simulink model "Sub2_2023"  (R2023b)
settings: Solver=FixedStepDiscrete  StartTime=0.0  StopTime=4.5  FixedStep=7.5e-05  RelTol=1e-3  EnableMultiTasking=on
undefined symbols (not defined in the file or in its folder): D1, D11, Delta
libraries: spsSeriesRLCBranchLib x41, spsLoadFlowBusLib x29, spsDistributedParametersLineLib x19, spsThreePhaseSeriesRLCLoadLib x15, spsThreePhaseTransformerTwoWindingsLib x13, spsThreePhaseParallelRLCLoadLib x11, spsThreePhaseVIMeasurementLib x11, spsSynchronousMachinepuStandardLib x7, spsExcitationSystemLib x7, spsHydraulicTurbineandGovernorLib x7, spsGenericPowerSystemStabilizerLib x7, spsMultiBandPowerSystemStabilizerLib x7
(part 3 of 5)

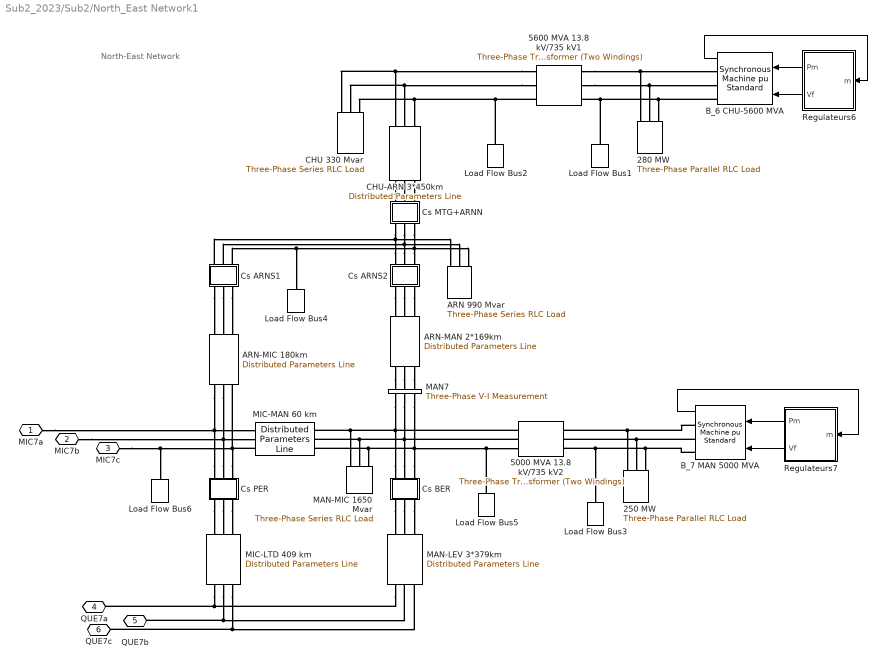
== system Sub2_2023/Sub2/North_East Network1 ==
  note: North-East Network
  250 MW : spsThreePhaseParallelRLCLoadLib/Three-Phase Parallel RLC Load  LConnTagsString=A|B|C  Configuration=Y (grounded)  NominalVoltage=(13800)*1  Vabc=[1e3 1e3 1e3]  Vabcp=[1e3 1e3 1e3]  NominalFrequency=60  UnbalancedPower=off  ActivePower=250000000  InductivePower=0  CapacitivePower=0  Pabc=[10e3 9e3 11e3]  QLabc=[100 90 110]  QCabc=[100 90 110]  Pabcp=[10e3 9e3 11e3]  QLabcp=[100 90 110]  QCabcp=[100 90 110]  Measurements=None  LoadType=constant PQ
  280 MW : spsThreePhaseParallelRLCLoadLib/Three-Phase Parallel RLC Load  LConnTagsString=A|B|C  Configuration=Y (grounded)  NominalVoltage=(13800)*1  Vabc=[1e3 1e3 1e3]  Vabcp=[1e3 1e3 1e3]  NominalFrequency=60  UnbalancedPower=off  ActivePower=280000000  InductivePower=0  CapacitivePower=0  Pabc=[10e3 9e3 11e3]  QLabc=[100 90 110]  QCabc=[100 90 110]  Pabcp=[10e3 9e3 11e3]  QLabcp=[100 90 110]  QCabcp=[100 90 110]  Measurements=None  LoadType=constant PQ
  5000 MVA 13.8 kV/735 kV2 : spsThreePhaseTransformerTwoWindingsLib/Three-Phase Transformer (Two Windings)  Winding1Connection=Delta (D1)  Winding2Connection=Yg  CoreType=Three single-phase transformers  SetSaturation=off  Hysteresis=off  DataFile='basic_model'  SetInitialFlux=off  Measurements=None  UNITS=pu  NominalPower=[ 5000e6 60 ]  Winding1="[ 13.8e3 0.002  0.0]"  Winding2=[ 735e3 0.002 0.12]  Rm=500  Lm=500  L0=0.5  Saturation="[ 0,0  ;  0.005,1.2  ;  1.0,1.4 ]"  InitialFluxes=[ 0.8 , -0.8 , 0.7 ]  BreakLoop=off  DiscreteSolver=Trapezoidal iterative  DataType=off  TransfoNumber=0
  5600 MVA 13.8 kV/735 kV1 : spsThreePhaseTransformerTwoWindingsLib/Three-Phase Transformer (Two Windings)  Winding1Connection=Delta (D1)  Winding2Connection=Yg  CoreType=Three single-phase transformers  SetSaturation=off  Hysteresis=off  DataFile='basic_model'  SetInitialFlux=off  Measurements=None  UNITS=pu  NominalPower=[ 5600e6 60 ]  Winding1="[ 13.8e3 0.002  0.0]"  Winding2=[ 735e3 0.002 0.12]  Rm=500  Lm=500  L0=0.5  Saturation="[ 0,0  ;  0.005,1.2  ;  1.0,1.4 ]"  InitialFluxes=[ 0.8 , -0.8 , 0.7 ]  BreakLoop=off  DiscreteSolver=Trapezoidal iterative  DataType=off  TransfoNumber=0
  ARN 990 Mvar : spsThreePhaseSeriesRLCLoadLib/Three-Phase Series RLC Load  LConnTagsString=A|B|C  Configuration=Y (grounded)  NominalVoltage=735e3  Vabc=[1e3 1e3 1e3]  Vabcp=[1e3 1e3 1e3]  NominalFrequency=60  UnbalancedPower=off  ActivePower=3300000  InductivePower=990e6  CapacitivePower=0  Pabc=[10e3 9e3 11e3]  QLabc=[100 90 110]  QCabc=[100 90 110]  Pabcp=[10e3 9e3 11e3]  QLabcp=[100 90 110]  QCabcp=[100 90 110]  Measurements=None  LoadType=constant Z
  ARN-MAN 2*169km : spsDistributedParametersLineLib/Distributed Parameters Line  Phases=3  Length=169  Frequency=60  Resistance="[0.01273  0.3864]/2"  Inductance="[0.9337e-3  4.1264e-3]/2"  Capacitance=[12.74e-9 7.751e-9]*2  x1=[-0.000975 1.7310716577648e-09 347873.977312542 -681165.145140991;-0.0009 1.66282026610766e-09 366991.883229433 -671058.367402292;-0.000825 1.59323964137178e-09 385816.421450034 -660415.155872229;-0.00075 1.52238540524399e-09 404332.543926518 -649244.018571252;-0.000675 1.45031419751651e-09 422525.449153882 -637553.885535596;-0.0006 1.37708363081009e-09 440380.594002048 -625354.101678744;-0.000525 1.30275224451929e-09 457883.705341419 -612654.419321249;-0.00045 1.227379458017e-09 475020.791452595 -599464.990394876;-0.000375 1.15102552315551e-09 491778.153211146 -585796.358327302;-0.0003 1.07375147610208e-09 508142.395038477 -571659.449613867;-0.000225 9.95619088547613e-10 524100.435610055 -557065.565083093;-0.00015 9.16690818327239e-10 539639.518312411 -542026.370862981;-7.5e-05 8.37029759492534e-10 554747.22144059 -526553.889055283]  x2=[-0.000975 1.53641947846113e-09 232985.418240288 -689450.364519062;-0.0009 1.49169542852533e-09 252383.458947623 -682588.200672253;-0.000825 1.44577894008767e-09 271579.748179473 -675180.386261777;-0.00075 1.39870671808647e-09 290558.940715937 -667232.842981129;-0.000675 1.35051639133576e-09 309305.864880893 -658751.923974807;-0.0006 1.30124648244541e-09 327805.534670003 -649744.408759702;-0.000525 1.25093637702673e-09 346043.16173029 -640217.497805657;-0.00045 1.19962629220823e-09 364004.167181727 -630178.806779522;-0.000375 1.14735724448663e-09 381674.19327137 -619636.360457307;-0.0003 1.09417101693894e-09 399039.114850723 -608598.586309297;-0.000225 1.04011012582169e-09 416085.050667168 -597074.307763262;-0.00015 9.85217786584077e-10 432798.374460424 -585072.737151144;-7.5e-05 9.29537879322206e-10 449165.725855173 -572603.46834486]  x3=[-0.000975 -3.38800758696293e-12 1583.75858462532 -1421.24992657805;-0.0009 -3.62113287945408e-12 1623.30400424475 -1375.90902523865;-0.000825 -3.85136349372659e-12 1661.55177948058 -1329.46824327658;-0.00075 -4.07851538695005e-12 1698.47133564649 -1281.96470474239;-0.000675 -4.30240697737656e-12 1734.03315981417 -1233.43638323794;-0.0006 -4.52285928949439e-12 1768.20882440548 -1183.92207156094;-0.000525 -4.73969609709827e-12 1800.97100991707 -1133.46135069455;-0.00045 -4.95274406416191e-12 1832.29352675911 -1082.09455816696;-0.000375 -5.16183288340019e-12 1862.15133619089 -1029.86275580616;-0.0003 -5.36679541241016e-12 1890.52057033639 -976.80769691581;-0.000225 -5.56746780728218e-12 1917.3785512639 -922.9717928982;-0.00015 -5.76368965357417e-12 1942.70380911441 -868.39807935129;-7.5e-05 -5.9553040945445e-12 1966.47609926427 -813.130181666682]  x4=[-0.000975 1.03362527745804e-11 1569.30174481215 -9115.59279820568;-0.0009 1.01548326150274e-11 1826.37892659032 -9067.58416140718;-0.000825 9.96529483765609e-12 2081.9961289991 -9012.32703656874;-0.00075 9.76779095606568e-12 2335.94901555798 -8949.86559539049;-0.000675 9.56247885183719e-12 2588.03458021503 -8880.24976859283;-0.0006 9.34952264832539e-12 2838.05130962692 -8803.53520600253;-0.000525 9.129092579461e-12 3085.79934424553 -8719.78323206715;-0.00045 8.90136485366839e-12 3331.08063808267 -8629.06079683322;-0.000375 8.66652151300721e-12 3573.69911702496 -8531.44042242736;-0.0003 8.42475028765076e-12 3813.46083557254 -8427.00014508323;-0.000225 8.17624444581736e-12 4050.17413187606 -8315.82345276054;-0.00015 7.92120263927471e-12 4283.64978094831 -8197.99921840608;-7.5e-05 7.65982874454068e-12 4513.70114592771 -8073.62162891002]  x5=0.000955765248222805  V1=ones(3,3)  V2=ones(3,3)  I1=ones(3,3)  I2=ones(3,3)  nHarmo=1  Measurements=None  Decoupling=on  VsMag0=[624500.542746028 624501.9043063 624500.043262054]  VrMag0=[594207.380493384 594208.101305747 594207.286862453]  VsAngle0=[18.1135948354144 -101.886530201481 138.113424134237]  VrAngle0=[9.73160889878888 -110.268441654022 129.731523430542]  IsMag0=[1744.35611857347 1744.39210598435 1744.37536737855]  IrMag0=[7582.44376493454 7582.43378992783 7582.40838117123]  IsAngle0=[39.1559168024549 -80.8440356055105 159.154916919419]  IrAngle0=[0.828149284031303 -119.172115933983 120.828081951977]
      settings: AttributesFormatString=\n  LibrarySourceBlock=sps_lib/Power Grid Elements/Distributed Parameters Line
  ARN-MIC 180km : spsDistributedParametersLineLib/Distributed Parameters Line  Phases=3  Length=180  Frequency=60  Resistance="[0.01273  0.3864]"  Inductance="[0.9337e-3  4.1264e-3]"  Capacitance=[12.74e-9 7.751e-9]  x1=[-0.00105 1.17550663706793e-09 336203.730988142 -674396.627298138;-0.000975 1.11045162417448e-09 355134.952563357 -664622.476598413;-0.0009 1.04450893324313e-09 373782.28469124 -654317.036859961;-0.000825 9.7773127785208e-10 392130.820979802 -643488.546093628;-0.00075 9.10172039037302e-10 410165.893889875 -632145.660429254;-0.000675 8.41885222620616e-10 427873.086460121 -620297.447196085;-0.0006 7.72925416038243e-10 445238.243831729 -607953.377674497;-0.000525 7.03347744704445e-10 462247.484563591 -595123.319524794;-0.00045 6.33207827945111e-10 478887.211728917 -581817.528899156;-0.000375 5.62561734536522e-10 495144.123784406 -568046.642243022;-0.0003 4.91465937884828e-10 511005.225203302 -553821.667792484;-0.000225 4.19977270882071e-10 526457.836863812 -539153.976774469;-0.00015 3.48152880474837e-10 541489.606184609 -524055.294316752;-7.5e-05 2.7605018198187e-10 556088.51699929 -508537.690075074]  x2=[-0.00105 4.32054145383614e-09 192165.57848684 -719334.039085178;-0.000975 4.26552520912623e-09 212424.764832694 -713613.931123558;-0.0009 4.20709916882887e-09 232514.142071749 -707323.371104057;-0.000825 4.14531003782672e-09 252417.651063218 -700467.387604106;-0.00075 4.08020720940571e-09 272119.381246546 -693051.461192015;-0.000675 4.01184272577075e-09 291603.583360071 -685081.520045889;-0.0006 3.94027123644407e-09 310854.682030743 -676563.935214738;-0.000525 3.86554995457915e-09 329857.288224836 -667505.515525552;-0.00045 3.78773861122544e-09 348596.211549708 -657913.502140431;-0.000375 3.70689940758025e-09 367056.472396768 -647795.562768113;-0.0003 3.62309696526611e-09 385223.313915946 -637159.785534523;-0.000225 3.53639827467318e-09 403082.213812094 -626014.672517248;-0.00015 3.44687264140818e-09 420618.895953885 -614369.132949109;-7.5e-05 3.35459163089256e-09 437819.341785936 -602232.476096253]  x3=[-0.00105 3.17397778533418e-12 149.001660749432 -364.5409355399;-0.000975 3.41695138621498e-12 159.247423691846 -360.183291874008;-0.0009 3.65719352843875e-12 169.365886680328 -355.537723195582;-0.000825 3.89451216611283e-12 179.348961170383 -350.607943101142;-0.00075 4.12871759034934e-12 189.188666845009 -345.397892381469;-0.000675 4.35962258091563e-12 198.877137994043 -339.91173587139;-0.0006 4.5870425558952e-12 208.406629801887 -334.153859120481;-0.000525 4.81079571923969e-12 217.769524538595 -328.128864887315;-0.00045 5.03070320609386e-12 226.958337649373 -321.841569460099;-0.000375 5.24658922577742e-12 235.965723737613 -315.296998806598;-0.0003 5.45828120230941e-12 244.784482436694 -308.500384556456;-0.000225 5.66560991236276e-12 253.407564165843 -301.457159819114;-0.00015 5.86840962053892e-12 261.828075765464 -294.172954840662;-7.5e-05 6.06651821185409e-12 270.039286007422 -286.653592503108]  x4=[-0.00105 3.98244780356522e-12 1187.65933351944 -4979.4651542716;-0.000975 3.61607808742167e-12 1327.95758028664 -4943.89904376789;-0.0009 3.24681773378287e-12 1467.19427808259 -4904.3808560128;-0.000825 2.87496192372567e-12 1605.25812322147 -4860.94218124095;-0.00075 2.50080791309503e-12 1742.03874957792 -4813.61774366432;-0.000675 2.12465479488231e-12 1877.42681681204 -4762.44537371424;-0.0006 1.74680326013487e-12 2011.3140977744 -4707.46597780026;-0.000525 1.36755535758826e-12 2143.59356502113 -4648.72350561027;-0.00045 9.87214252213096e-13 2274.15947637007 -4586.26491497776;-0.000375 6.06083982869597e-13 2402.9074594294 -4520.14013434441;-0.0003 2.24469219263587e-13 2529.73459503138 -4450.40202284814;-0.000225 -1.57324981601807e-13 2654.53949950433 -4377.10632806823;-0.00015 -5.38993419284062e-13 2777.22240571719 -4300.31164146164;-7.5e-05 -9.20230993873817e-13 2897.68524283186 -4220.07935152584]  x5=0.00101797482059234  V1=ones(3,3)  V2=ones(3,3)  I1=ones(3,3)  I2=ones(3,3)  nHarmo=1  Measurements=None  Decoupling=on  VsMag0=[615273.936100198 615275.237959109 615273.425867188]  VrMag0=[607930.231676026 607930.976808573 607930.152147035]  VsAngle0=[19.1774103741833 -100.822714483785 139.17724295487]  VrAngle0=[7.63692875074031 -112.363120449614 127.636843332411]  IsMag0=[322.896150602072 322.910343515583 322.909058922829]  IrMag0=[4197.50413399039 4197.49907033644 4197.4882687283]  IsAngle0=[14.9112658693506 -105.087543385411 134.909680310663]  IrAngle0=[6.09512812442481 -113.905082032172 126.095082904961]
      settings: AttributesFormatString=\n  LibrarySourceBlock=sps_lib/Power Grid Elements/Distributed Parameters Line
  "B_6 CHU-5600 MVA " : spsSynchronousMachinepuStandardLib/Synchronous Machine pu Standard  PresetModel=No  MechanicalLoad=Mechanical power Pm  ShowDetailedParameters=on  RotorType=Salient-pole  Units=per unit standard parameters  MeasurementBus=off  NominalParameters="[ 5600E6  13800   60 ]"  Reactances1=[ 31 32 33 34 35 36 37 ]  Reactances2=[ 1.305, 0.296, 0.252, 0.474, 0.243, 0.18 ]  dAxisTimeConstants=Short-circuit  qAxisTimeConstants=Open-circuit  TimeConstants1=[]  TimeConstants2=[]  TimeConstants3=[]  TimeConstants4=[]  TimeConstants5=[ 1.01, 0.053, 0.1 ]  TimeConstants6=[]  TimeConstants7=[]  TimeConstants8=[]  StatorResistance=2.8544e-3  Mechanical="[ 4.0 0  32]"  PolePairs=32  InitialConditions=[0 -61.7964 0.894782 0.894782 0.894782 8.48442 -111.516 128.484 1.31361]  SetSaturation=off  Saturation=[0.6404,0.7127,0.8441,0.9214,0.9956,1.082,1.19,1.316,1.457;0.7,0.7698,0.8872,0.9466,0.9969,1.046,1.1,1.151,1.201]  LoadFlowParameters=[1 5000000000 0 0 0]  TsPowergui=0  TsBlock=-1  IterativeModel=Trapezoidal non iterative  IterativeDiscreteModel=Trapezoidal non iterative  BusType=PV  Pref=5000000000  Qref=0  Qmin=-Inf  Qmax=Inf  PLF=0  QLF=0
  B_7 MAN 5000 MVA : spsSynchronousMachinepuStandardLib/Synchronous Machine pu Standard  PresetModel=No  MechanicalLoad=Mechanical power Pm  ShowDetailedParameters=on  RotorType=Salient-pole  Units=per unit standard parameters  MeasurementBus=off  NominalParameters="[ 5000E6  13800   60 ]"  Reactances1=[ 31 32 33 34 35 36 37 ]  Reactances2=[ 1.305, 0.296, 0.252, 0.474, 0.243, 0.18 ]  dAxisTimeConstants=Short-circuit  qAxisTimeConstants=Open-circuit  TimeConstants1=[]  TimeConstants2=[]  TimeConstants3=[]  TimeConstants4=[]  TimeConstants5=[ 1.01, 0.053, 0.1 ]  TimeConstants6=[]  TimeConstants7=[]  TimeConstants8=[]  StatorResistance=2.8544e-3  Mechanical="[ 3.7 0  32]"  PolePairs=32  InitialConditions=[0 -81.9543 0.907703 0.907703 0.907703 -8.76021 -128.76 111.24 1.25655]  SetSaturation=off  Saturation=[0.6404,0.7127,0.8441,0.9214,0.9956,1.082,1.19,1.316,1.457;0.7,0.7698,0.8872,0.9466,0.9969,1.046,1.1,1.151,1.201]  LoadFlowParameters=[1 4500000000 0 0 0]  TsPowergui=0  TsBlock=-1  IterativeModel=Trapezoidal non iterative  IterativeDiscreteModel=Trapezoidal non iterative  BusType=PV  Pref=4500000000  Qref=0  Qmin=-Inf  Qmax=Inf  PLF=0  QLF=0
  CHU 330 Mvar : spsThreePhaseSeriesRLCLoadLib/Three-Phase Series RLC Load  LConnTagsString=A|B|C  Configuration=Y (grounded)  NominalVoltage=735e3  Vabc=[1e3 1e3 1e3]  Vabcp=[1e3 1e3 1e3]  NominalFrequency=60  UnbalancedPower=off  ActivePower=1100000  InductivePower=330e6  CapacitivePower=0  Pabc=[10e3 9e3 11e3]  QLabc=[100 90 110]  QCabc=[100 90 110]  Pabcp=[10e3 9e3 11e3]  QLabcp=[100 90 110]  QCabcp=[100 90 110]  Measurements=None  LoadType=constant Z
  CHU-ARN 3*450km : spsDistributedParametersLineLib/Distributed Parameters Line  Phases=3  Length=450  Frequency=60  Resistance="[0.01273  0.3864]/3"  Inductance="[0.9337e-3  4.1264e-3]/3"  Capacitance=[12.74e-9 7.751e-9]*3  x1=[-0.00255 1.80867377993606e-09 0 0;-0.002475 1.72308488593625e-09 0 0;-0.0024 1.6361185842427e-09 0 0;-0.002325 1.54784439438636e-09 0 0;-0.00225 1.45833288140396e-09 0 0;-0.002175 1.36765559942941e-09 0 0;-0.0021 1.2758850344945e-09 0 0;-0.002025 1.18309454658472e-09 0 0;-0.00195 1.08935831099635e-09 0 0;-0.001875 9.94751259041912e-10 0 0;-0.0018 8.993490181512e-10 0 0;-0.001725 8.03227851415879e-10 0 0;-0.00165 7.06464596625934e-10 0 0;-0.001575 6.09136604846718e-10 336692.12965357 -649852.524072933;-0.0015 5.1132167858569e-10 354929.318552013 -640074.408280607;-0.001425 4.13098009598284e-10 372882.782383807 -629784.626799769;-0.00135 3.14544116382617e-10 390538.16942466 -618991.405124295;-0.001275 2.15738781413e-10 407881.36622831 -607703.37119045;-0.0012 1.16760988162435e-10 424898.508908591 -595929.54847985;-0.001125 1.76898579644369e-11 441575.994222016 -583679.348806222;-0.00105 -8.13954132353542e-11 457900.490441999 -570962.564791752;-0.000975 -1.80415618187197e-10 473858.948016035 -557789.362039008;-0.0009 -2.79291601654312e-10 489438.609997312 -544170.271004713;-0.000825 -3.7794432368837e-10 504627.022242419 -530116.178581862;-0.00075 -4.76294922812813e-10 519412.043366998 -515638.319396901;-0.000675 -5.74264779063516e-10 533781.85445138 -500748.266828946;-0.0006 -6.71775576836382e-10 547724.96848845 -485457.923758193;-0.000525 -7.68749367491635e-10 561230.239566184 -469779.513050943;-0.00045 -8.65108631664776e-10 574286.871777518 -453725.567788827;-0.000375 -9.60776341234369e-10 586884.427850438 -437308.921250055;-0.0003 -1.05567602089715e-09 599012.837491367 -420542.696650687;-0.000225 -1.14973180930121e-09 610662.405435208 -403440.296654135;-0.00015 -1.24286851968841e-09 621823.819195594 -386015.392657282;-7.5e-05 -1.33501169999749e-09 632488.156509137 -368281.913861772]  x2=[-0.00255 2.55703265416158e-09 0 0;-0.002475 2.53163349239611e-09 0 0;-0.0024 2.50421058155211e-09 0 0;-0.002325 2.47478584308493e-09 0 0;-0.00225 2.44338279868027e-09 0 0;-0.002175 2.41002655145137e-09 0 0;-0.0021 2.37474376587187e-09 0 0;-0.002025 2.33756264646073e-09 0 0;-0.00195 2.29851291523592e-09 0 0;-0.001875 2.2576257879551e-09 0 0;-0.0018 2.21493394916222e-09 0 0;-0.001725 2.17047152606001e-09 0 0;-0.00165 2.12427406122919e-09 0 0;-0.001575 2.07637848421631e-09 24661.2186380129 -733238.396737066;-0.0015 2.0268230820128e-09 45380.4401578333 -732248.159297928;-0.001425 1.97564746844896e-09 66063.3852481355 -730672.573884019;-0.00135 1.92289255252726e-09 86693.5202790741 -728512.899994213;-0.001275 1.86860050572032e-09 107254.353836357 -725770.864038773;-0.0012 1.81281472825965e-09 127729.44990423 -722448.657959287;-0.001125 1.75557981444221e-09 148102.441004175 -718548.937476463;-0.00105 1.69694151698237e-09 168357.041278825 -714074.819967188;-0.000975 1.63694671043793e-09 188477.059510626 -709029.881972542;-0.0009 1.5756433537393e-09 208446.412064849 -703418.156338769;-0.000825 1.51308045185183e-09 228249.135746606 -697244.128993477;-0.00075 1.44930801660206e-09 247869.400561575 -690512.73535966;-0.000675 1.38437702669898e-09 267291.522370264 -683229.356410397;-0.0006 1.31833938698243e-09 286499.975425668 -675399.814367378;-0.000525 1.2512478869312e-09 305479.404784313 -667030.368046718;-0.00045 1.18315615846389e-09 324214.638580765 -658127.707855748;-0.000375 1.1141186330664e-09 342690.700155786 -648698.95044481;-0.0003 1.04419049828023e-09 360892.820028447 -638751.633018313;-0.000225 9.73427653586374e-10 378806.447702621 -628293.707309608;-0.00015 9.01886665720188e-10 396417.263298435 -617333.533224497;-7.5e-05 8.29624723452754e-10 413711.188999357 -605879.872158446]  x3=[-0.00255 4.79707758720459e-12 0 0;-0.002475 4.73527209386888e-12 0 0;-0.0024 4.66968129647343e-12 0 0;-0.002325 4.60035762729809e-12 0 0;-0.00225 4.52735650262333e-12 0 0;-0.002175 4.45073627843124e-12 0 0;-0.0021 4.37055820375673e-12 0 0;-0.002025 4.28688637172591e-12 0 0;-0.00195 4.1997876683211e-12 0 0;-0.001875 4.10933171891314e-12 0 0;-0.0018 4.01559083260396e-12 0 0;-0.001725 3.9186399444238e-12 0 0;-0.00165 3.81855655542927e-12 0 0;-0.001575 3.7154206707502e-12 -336.540930617868 -2064.60581281028;-0.0015 3.60931473563478e-12 -278.039507495116 -2073.29664774071;-0.001425 3.50032356954406e-12 -219.315823844219 -2080.33012105345;-0.00135 3.38853429834859e-12 -160.416822479385 -2085.70061029753;-0.001275 3.27403628468133e-12 -101.389586361122 -2089.40382238603;-0.0012 3.15692105650254e-12 -42.2813009588338 -2091.43679702786;-0.001125 3.03728223393369e-12 16.8607834685153 -2091.7979090942;-0.00105 2.91521545441901e-12 75.9893896435381 -2090.4868699176;-0.000975 2.79081829627436e-12 135.057251063157 -2087.50472752271;-0.0009 2.66419020068462e-12 194.01714978272 -2082.85386578852;-0.000825 2.53543239221193e-12 252.82195416131 -2076.53800254276;-0.00075 2.40464779787832e-12 311.424656538048 -2068.56218658987;-0.000675 2.27194096488743e-12 369.778410809307 -2058.93279367507;-0.0006 2.13741797705108e-12 427.836569876765 -2047.65752138774;-0.000525 2.00118636998746e-12 485.552722936382 -2034.74538300803;-0.00045 1.86335504515885e-12 542.880732578489 -2020.20670030178;-0.000375 1.72403418281743e-12 599.774771669327 -2004.05309526952;-0.0003 1.58333515392887e-12 656.189359984554 -1986.29748085593;-0.000225 1.4413704311441e-12 712.079400565444 -1966.95405062752;-0.00015 1.29825349889039e-12 767.400215768702 -1946.03826742645;-7.5e-05 1.1540987626536e-12 822.107582981091 -1923.56685100977]  x4=[-0.00255 1.90509802475781e-11 0 0;-0.002475 1.89178495284245e-11 0 0;-0.0024 1.87695961698107e-11 0 0;-0.002325 1.86063386832032e-11 0 0;-0.00225 1.84282075741389e-11 0 0;-0.002175 1.82353452379009e-11 0 0;-0.0021 1.80279058456898e-11 0 0;-0.002025 1.78060552213818e-11 0 0;-0.00195 1.75699707089717e-11 0 0;-0.001875 1.73198410308064e-11 0 0;-0.0018 1.70558661367235e-11 0 0;-0.001725 1.67782570442144e-11 0 0;-0.00165 1.64872356697402e-11 0 0;-0.001575 1.61830346513347e-11 -291.743024303928 -14207.2379327624;-0.0015 1.58658971626376e-11 110.022151992647 -14209.8063832468;-0.001425 1.55360767185051e-11 511.699378264315 -14201.0157319257;-0.00135 1.51938369723538e-11 912.967559882261 -14180.8730059114;-0.001275 1.48394515054003e-11 1313.50592920171 -14149.3943069907;-0.0012 1.44732036079646e-11 1712.99430197867 -14106.6047987541;-0.001125 1.40953860530121e-11 2111.11333332032 -14052.5386864796;-0.00105 1.37063008621155e-11 2507.54477296443 -13987.2391897902;-0.000975 1.33062590640231e-11 2901.97171968375 -13910.7585081044;-0.0009 1.28955804460276e-11 3294.07887461201 -13823.157778909;-0.000825 1.24745932983325e-11 3683.55279328901 -13724.5070288866;-0.00075 1.20436341516223e-11 4070.0821362233 -13614.8851179372;-0.000675 1.16030475080452e-11 4453.35791777224 -13494.3796761393;-0.0006 1.11531855658227e-11 4833.07375314037 -13363.0870336992;-0.000525 1.06944079377084e-11 5208.92610329875 -13221.1121439465;-0.00045 1.02270813635185e-11 5580.61451762939 -13068.5684994357;-0.000375 9.75157941696631e-12 5947.84187410091 -12905.5780412222;-0.0003 9.26828220703232e-12 6310.3146167833 -12732.2710613846;-0.000225 8.77757607411151e-12 6667.74299051209 -12548.7860988707;-0.00015 8.27985328117847e-12 7019.84127251415 -12355.2698287523;-7.5e-05 7.77551170021847e-12 7366.32800081013 -12151.8769449748]  x5=0.00254493705148084  V1=ones(3,3)  V2=ones(3,3)  I1=ones(3,3)  I2=ones(3,3)  nHarmo=1  Measurements=None  Decoupling=on  VsMag0=[597589.636778476 597591.191031021 597588.179734199]  VrMag0=[599025.218159165 599025.681050673 599025.146419465]  VsAngle0=[31.4089201475902 -88.5913271983155 151.408667420066]  VrAngle0=[5.9463220799337 -114.053711405448 125.946266994119]  IsMag0=[1726.12548309379 1726.16866029094 1726.16794416809]  IrMag0=[11726.067575369 11726.0492062877 11726.0164561764]  IsAngle0=[-5.23898774455876 -125.238187761817 114.760171100695]  IrAngle0=[2.84375678806129 -117.156479810906 122.843716218945]
      settings: AttributesFormatString=\n  LibrarySourceBlock=sps_lib/Power Grid Elements/Distributed Parameters Line
  "Cs ARNS1 " : Subsystem  mask{Xc=25}
      mask prompts: Xc "Condensator Reactance at  60Hz  (ohm):"
      mask help: Series Compensation
      mask init:
      | Cs=1/Xc/(2*pi*60);
      mask Display: disp('Cs')
  Cs ARNS2 : Subsystem  mask{Xc=25/2}
      mask prompts: Xc "Condensator Reactance at  60Hz  (ohm):"
      mask help: Series Compensation
      mask init:
      | Cs=1/Xc/(2*pi*60);
      mask Display: disp('Cs')
  Cs BER : Subsystem  mask{Xc=22/3}
      mask prompts: Xc "Condensator Reactance at  60Hz  (ohm):"
      mask help: Series Compensation
      mask init:
      | Cs=1/Xc/(2*pi*60);
      mask Display: disp('Cs')
  "Cs MTG+ARNN " : Subsystem  mask{Xc=(30+25)/3}
      mask prompts: Xc "Condensator Reactance at  60Hz  (ohm):"
      mask help: Series Compensation
      mask init:
      | Cs=1/Xc/(2*pi*60);
      mask Display: disp('Cs')
  "Cs PER " : Subsystem  mask{Xc=22}
      mask prompts: Xc "Condensator Reactance at  60Hz  (ohm):"
      mask help: Series Compensation
      mask init:
      | Cs=1/Xc/(2*pi*60);
      mask Display: disp('Cs')
  Load Flow Bus1 : spsLoadFlowBusLib/Load Flow Bus  LConnTagsString=a  Phases=single  Connectors=on one side  ID=CHU_13.8  Vbase=13.8e3  Vref=1  Vangle=0  VLF=1  VLFb=1  VLFc=1  angleLF=4.726  angleLFb=0  angleLFc=0
      settings: AttributesFormatString=%<ID>\n%<Vbase>V\n%<VLF>pu\n%<angleLF>deg.
  Load Flow Bus2 : spsLoadFlowBusLib/Load Flow Bus  LConnTagsString=a  Phases=single  Connectors=on one side  ID=CHU7  Vbase=735e3  Vref=1  Vangle=0  VLF=1.009  VLFb=1  VLFc=1  angleLF=28.97  angleLFb=0  angleLFc=0
      settings: AttributesFormatString=%<ID>\n%<Vbase>V\n%<VLF>pu\n%<angleLF>deg.
  Load Flow Bus3 : spsLoadFlowBusLib/Load Flow Bus  LConnTagsString=a  Phases=single  Connectors=on one side  ID=MAN_13.8  Vbase=13.8e3  Vref=1  Vangle=0  VLF=1  VLFb=1  VLFc=1  angleLF=-16.23  angleLFb=0  angleLFc=0
      settings: AttributesFormatString=%<ID>\n%<Vbase>V\n%<VLF>pu\n%<angleLF>deg.
  Load Flow Bus4 : spsLoadFlowBusLib/Load Flow Bus  LConnTagsString=a  Phases=single  Connectors=on one side  ID=ARN7  Vbase=735e3  Vref=1  Vangle=0  VLF=1.054  VLFb=1  VLFc=1  angleLF=12.72  angleLFb=0  angleLFc=0
      settings: AttributesFormatString=%<ID>\n%<Vbase>V\n%<VLF>pu\n%<angleLF>deg.
  Load Flow Bus5 : spsLoadFlowBusLib/Load Flow Bus  LConnTagsString=a  Phases=single  Connectors=on one side  ID=MAN7  Vbase=735e3  Vref=1  Vangle=0  VLF=1.016  VLFb=1  VLFc=1  angleLF=7.996  angleLFb=0  angleLFc=0
      settings: AttributesFormatString=%<ID>\n%<Vbase>V\n%<VLF>pu\n%<angleLF>deg.
  Load Flow Bus6 : spsLoadFlowBusLib/Load Flow Bus  LConnTagsString=a  Phases=single  Connectors=on one side  ID=MIC7  Vbase=735e3  Vref=1  Vangle=0  VLF=1.041  VLFb=1  VLFc=1  angleLF=5.981  angleLFb=0  angleLFc=0
      settings: AttributesFormatString=%<ID>\n%<Vbase>V\n%<VLF>pu\n%<angleLF>deg.
  MAN-LEV 3*379km : spsDistributedParametersLineLib/Distributed Parameters Line  Phases=3  Length=379  Frequency=60  Resistance="[0.01273  0.3864]/3"  Inductance="[0.9337e-3  4.1264e-3]/3"  Capacitance=[12.74e-9 7.751e-9]*3  x1=[-0.002175 3.17741333780928e-09 -30838.3336725922 -721772.968424234;-0.0021 3.13733455956081e-09 -10421.0500052849 -722356.32852349;-0.002025 3.09474784406825e-09 10004.5640899494 -722362.248026147;-0.00195 3.04968723450037e-09 30422.1806897252 -721790.722200244;-0.001875 3.00218875161901e-09 50815.4782637324 -720642.207914784;-0.0018 2.95229036498464e-09 71168.1547219185 -718917.623274511;-0.001725 2.90003196260405e-09 91463.9404461292 -716618.346886002;-0.00165 2.84545531904454e-09 111686.611295792 -713746.21675562;-0.001575 2.7886040620399e-09 131820.001577248 -710303.528820247;-0.0015 2.72952363761515e-09 151848.016966357 -706293.035111943;-0.001425 2.6682612737576e-09 171754.647374056 -701717.941558017;-0.00135 2.60486594266357e-09 191523.979744577 -696581.905418254;-0.001275 2.53938832159076e-09 211140.210776106 -690889.03236136;-0.0012 2.47188075234762e-09 230587.659553695 -684643.873182954;-0.001125 2.4023971994521e-09 249850.780084345 -677851.420167727;-0.00105 2.33099320699324e-09 268914.173724241 -670517.103098692;-0.000975 2.2577258542301e-09 287762.601488187 -662646.784916697;-0.0009 2.18265370996346e-09 306380.996231419 -654246.757033674;-0.000825 2.10583678571679e-09 324754.47469405 -645323.73430339;-0.00075 2.02733648776401e-09 342868.34939852 -635884.849653689;-0.000675 1.94721556804219e-09 360708.140390543 -625937.648384538;-0.0006 1.86553807398868e-09 378259.586814157 -615490.082136436;-0.000525 1.78236929734252e-09 395508.658311638 -604550.502533988;-0.00045 1.69777572195122e-09 412441.56623915 -593127.654509748;-0.000375 1.61182497062463e-09 429044.774689178 -581230.669313649;-0.0003 1.52458575107827e-09 445305.011310925 -568869.057213629;-0.000225 1.43612780100945e-09 461209.277920025 -556052.699893261;-0.00015 1.34652183234999e-09 476744.860889094 -542791.84255249;-7.5e-05 1.25583947474023e-09 491899.341310809 -529097.085717776]  x2=[-0.002175 1.35323407421467e-08 -379192.17523209 -624794.196144462;-0.0021 1.35998273688356e-08 -361377.320734367 -635264.4515137;-0.002025 1.36564425016101e-08 -343273.586735707 -645226.88620027;-0.00195 1.37021408831995e-08 -324895.445084072 -654673.536386314;-0.001875 1.37368859830166e-08 -306257.586984704 -663596.850564212;-0.0018 1.37606500263603e-08 -287374.911256199 -671989.695573141;-0.001725 1.3773414016618e-08 -268262.512420618 -679845.362301216;-0.00165 1.3775167750451e-08 -248935.668637164 -687157.57104865;-0.001575 1.37659098259515e-08 -229409.829489044 -693920.476547652;-0.0015 1.37456476437626e-08 -209700.603633318 -700128.67263504;-0.001425 1.37143974011628e-08 -189823.746323575 -705777.196573853;-0.00135 1.36721840791177e-08 -169795.146815422 -710861.533020477;-0.001275 1.36190414223113e-08 -149630.815664857 -715377.617634151;-0.0012 1.35550119121701e-08 -129346.871929678 -719321.840325932;-0.001125 1.34801467329051e-08 -108959.530284152 -722691.048144551;-0.00105 1.33945057305949e-08 -88485.088057253 -725482.547796826;-0.000975 1.32981573653464e-08 -67939.9122048288 -727694.107800648;-0.0009 1.31911786565688e-08 -47340.4262261034 -729323.960268787;-0.000825 1.30736551214049e-08 -26703.0970349858 -730370.802322118;-0.00075 1.29456807063705e-08 -6044.42179666949 -730833.797131121;-0.000675 1.28073577122551e-08 14619.0852599484 -730712.574584829;-0.0006 1.26587967123436e-08 35270.9060434889 -730007.231586691;-0.000525 1.25001164640264e-08 55894.5318044012 -728718.331977109;-0.00045 1.2331443813866e-08 76473.4763318042 -726846.906082708;-0.000375 1.21529135961982e-08 96991.2891323108 -724394.449892715;-0.0003 1.19646685253474e-08 117431.568580302 -721362.923863085;-0.000225 1.1766859081543e-08 137777.975029133 -717754.751349341;-0.00015 1.15596433906279e-08 158014.243872799 -713572.816669385;-7.5e-05 1.13431870976547e-08 178124.198547612 -708820.462797813]  x3=[-0.002175 3.13707257052003e-12 -359.273937220793 349.814819579099;-0.0021 4.73487591554552e-12 -369.020063583212 339.517457525765;-0.002025 6.32889427321016e-12 -378.471200953 328.948690411676;-0.00195 7.91785340962812e-12 -387.619794235549 318.116966747556;-0.001875 9.50048313517765e-12 -396.458530185368 307.030945247571;-0.0018 1.10755183198712e-11 -404.980343252175 295.699487907686;-0.001725 1.26416999046809e-11 -413.178421228994 284.131652921521;-0.00165 1.41977759080113e-11 -421.046210697724 272.336687439371;-0.001575 1.57425024265142e-11 -428.577422267846 260.324020176173;-0.0015 1.72746446294456e-11 -435.766035604061 248.103253874337;-0.001425 1.87929777457712e-11 -442.606304238858 235.684157627461;-0.00135 2.0296288043229e-11 -449.09276016615 223.076659071066;-0.001275 2.17833737985687e-11 -455.220218212315 210.290836446597;-0.0012 2.32530462581906e-11 -460.983780181144 197.336910545031;-0.001125 2.47041305884172e-11 -466.378838769385 184.225236536531;-0.00105 2.61354668146373e-11 -471.401081249749 170.966295692684;-0.000975 2.75459107485719e-11 -476.04649291844 157.570687007932;-0.0009 2.89343349029206e-11 -480.311360304448 144.049118726899;-0.000825 3.02996293926581e-11 -484.192274138038 130.412399784381;-0.00075 3.1640702822259e-11 -487.686132076073 116.671431164851;-0.000675 3.29564831581427e-11 -490.790141181974 102.837197188382;-0.0006 3.4245918585641e-11 -493.501820158356 88.9207567299414;-0.000525 3.5507978349802e-11 -495.819001330534 74.9332343791045;-0.00045 3.67416535793604e-11 -497.739832379333 60.8858115472219;-0.000375 3.79459580932137e-11 -499.262777821803 46.7897175291726;-0.0003 3.91199291887599e-11 -500.386620238659 32.6562205268371;-0.000225 4.02626284114675e-11 -501.110461247468 18.4966186414694;-0.00015 4.13731423050619e-11 -501.433722220804 4.32223084216752;-7.5e-05 4.2450583141728e-11 -501.356144748789 -9.85561208233727]  x4=[-0.002175 5.03958179901784e-11 -7842.63207577855 -13937.1348474411;-0.0021 4.96187071523364e-11 -7445.48599612156 -14153.2795346858;-0.002025 4.88019318791884e-11 -7042.38810887903 -14358.110306823;-0.00195 4.79461450883909e-11 -6633.6606443344 -14551.4634252674;-0.001875 4.70520308828103e-11 -6219.63033296911 -14733.1843264945;-0.0018 4.61203040036621e-11 -5800.62814427918 -14903.1277455962;-0.001725 4.51517092591578e-11 -5376.98902220329 -15061.1578324036;-0.00165 4.4147020929116e-11 -4949.05161737375 -15207.1482600833;-0.001575 4.31070421460156e-11 -4517.15801640431 -15340.982326121;-0.0015 4.20326042529835e-11 -4081.6534684314 -15462.5530456121;-0.001425 4.09245661392319e-11 -3642.8861091272 -15571.7632367835;-0.00135 3.97838135534756e-11 -3201.2066824054 -15668.5255986794;-0.001275 3.86112583958773e-11 -2756.96826004179 -15752.7627809482;-0.0012 3.74078379890894e-11 -2310.52595943413 -15824.4074456753;-0.001125 3.61745143289722e-11 -1862.23665972673 -15883.4023212118;-0.00105 3.4912273315589e-11 -1412.45871652673 -15929.700247957;-0.000975 3.36221239650931e-11 -961.551675440071 -15963.2642160566;-0.0009 3.23050976031351e-11 -509.875984656302 -15984.0673949879;-0.000825 3.09622470404379e-11 -57.7927068117633 -15992.0931550082;-0.00075 2.95946457311947e-11 394.336769638342 -15987.3350804476;-0.000675 2.82033869149673e-11 846.151019308355 -15969.796974838;-0.0006 2.67895827427664e-11 1297.28886880008 -15939.4928578729;-0.000525 2.53543633880152e-11 1747.38968541926 -15896.4469541996;-0.00045 2.38988761431065e-11 2196.09366545989 -15840.693674055;-0.000375 2.2424284502274e-11 2643.0421218257 -15772.277585758;-0.0003 2.09317672315134e-11 3087.87777075923 -15691.2533800829;-0.000225 1.94225174262948e-11 3530.24501744892 -15597.68582654;-0.00015 1.789774155782e-11 3969.79024028623 -15491.6497216;-7.5e-05 1.63586585085886e-11 4406.16207354528 -15373.2298289027]  x5=0.00214340253891386  V1=ones(3,3)  V2=ones(3,3)  I1=ones(3,3)  I2=ones(3,3)  nHarmo=1  Measurements=None  Decoupling=on  VsMag0=[589863.022608764 589863.802580153 589862.857709211]  VrMag0=[596743.737336293 596743.911083344 596743.706580488]  VsAngle0=[14.5334919446 -105.466570291728 134.533395214777]  VrAngle0=[-14.2738568821762 -134.273869923445 105.726122150017]  IsMag0=[413.109398330454 413.092934230172 413.107596303835]  IrMag0=[13174.4675205298 13174.4678533397 13174.4493337448]  IsAngle0=[-117.256344753859 122.744684998139 2.74614766468251]  IrAngle0=[-12.387010258645 -132.387102424569 107.612942404914]
      settings: AttributesFormatString=\n  LibrarySourceBlock=sps_lib/Power Grid Elements/Distributed Parameters Line
  MAN-MIC 1650 Mvar : spsThreePhaseSeriesRLCLoadLib/Three-Phase Series RLC Load  LConnTagsString=A|B|C  Configuration=Y (grounded)  NominalVoltage=735e3  Vabc=[1e3 1e3 1e3]  Vabcp=[1e3 1e3 1e3]  NominalFrequency=60  UnbalancedPower=off  ActivePower=5500000  InductivePower=1650e6  CapacitivePower=0  Pabc=[10e3 9e3 11e3]  QLabc=[100 90 110]  QCabc=[100 90 110]  Pabcp=[10e3 9e3 11e3]  QLabcp=[100 90 110]  QCabcp=[100 90 110]  Measurements=None  LoadType=constant Z
  MAN7 : spsThreePhaseVIMeasurementLib/Three-Phase V-I Measurement  VoltageMeasurement=no  SetLabelV=on  LabelV=Vabc_MAN7  Vpu=on  VpuLL=off  CurrentMeasurement=no  SetLabelI=on  LabelI=Iabc_MAN7  Ipu=on  Pbase=100e6  Vbase=735e3  OutputType=Magnitude  PhasorSimulation=off  PSBequivalent=0
  MIC-LTD 409 km : spsDistributedParametersLineLib/Distributed Parameters Line  Phases=3  Length=409  Frequency=60  Resistance="[0.01273  0.3864]"  Inductance="[0.9337e-3  4.1264e-3]"  Capacitance=[12.74e-9 7.751e-9]  x1=[-0.002325 4.42673995818441e-09 0 0;-0.00225 4.43640389057819e-09 0 0;-0.002175 4.44252142958111e-09 0 0;-0.0021 4.44508768492607e-09 0 0;-0.002025 4.44410060518782e-09 0 0;-0.00195 4.43956097942281e-09 0 0;-0.001875 4.43147243653841e-09 0 0;-0.0018 4.41984144239204e-09 0 0;-0.001725 4.40467729462246e-09 0 0;-0.00165 4.38599211521739e-09 0 0;-0.001575 4.36380084082334e-09 0 0;-0.0015 4.33812121080553e-09 0 0;-0.001425 4.30897375306728e-09 138503.934059122 -724390.238526883;-0.00135 4.27638176764033e-09 158927.516108478 -720185.156864022;-0.001275 4.24037130805918e-09 179224.05393313 -715404.370205966;-0.0012 4.20097116053421e-09 199377.322791287 -710051.700240421;-0.001125 4.15821282094053e-09 219371.21246818 -704131.425809859;-0.00105 4.11213046964058e-09 239189.740154319 -697648.279491077;-0.000975 4.0627609441609e-09 258817.063221903 -690607.443812047;-0.0009 4.01014370974479e-09 278237.491889183 -683014.547109081;-0.000825 3.95432082780436e-09 297435.501762622 -674875.659027629;-0.00075 3.89533692229733e-09 316395.746246868 -666197.285670295;-0.000675 3.83323914405526e-09 335103.068812581 -656986.364395956;-0.0006 3.76807713309197e-09 353542.515112335 -647250.258274147;-0.000525 3.69990297892199e-09 371699.344934889 -636996.750199135;-0.00045 3.62877117892107e-09 389559.043988294 -626234.036668391;-0.000375 3.55473859476179e-09 407107.335502387 -614970.721230436;-0.0003 3.47786440695918e-09 424330.191641431 -603215.807607297;-0.000225 3.39821006756276e-09 441213.844717747 -590978.692497069;-0.00015 3.31583925103268e-09 457744.798197393 -578269.158062335;-7.5e-05 3.23081780333937e-09 473909.83748909 -565097.364110461]  x2=[-0.002325 1.3364977445514e-08 0 0;-0.00225 1.34540365693203e-08 0 0;-0.002175 1.35323407421467e-08 0 0;-0.0021 1.35998273688356e-08 0 0;-0.002025 1.36564425016101e-08 0 0;-0.00195 1.37021408831995e-08 0 0;-0.001875 1.37368859830166e-08 0 0;-0.0018 1.37606500263603e-08 0 0;-0.001725 1.3773414016618e-08 0 0;-0.00165 1.3775167750451e-08 0 0;-0.001575 1.37659098259515e-08 0 0;-0.0015 1.37456476437626e-08 0 0;-0.001425 1.37143974011628e-08 -189823.746323575 -705777.196573853;-0.00135 1.36721840791177e-08 -169795.146815422 -710861.533020477;-0.001275 1.36190414223113e-08 -149630.815664857 -715377.617634151;-0.0012 1.35550119121701e-08 -129346.871929678 -719321.840325932;-0.001125 1.34801467329051e-08 -108959.530284152 -722691.048144551;-0.00105 1.33945057305949e-08 -88485.088057253 -725482.547796826;-0.000975 1.32981573653464e-08 -67939.9122048288 -727694.107800648;-0.0009 1.31911786565688e-08 -47340.4262261034 -729323.960268787;-0.000825 1.30736551214049e-08 -26703.0970349858 -730370.802322118;-0.00075 1.29456807063705e-08 -6044.42179666949 -730833.797131121;-0.000675 1.28073577122551e-08 14619.0852599484 -730712.574584829;-0.0006 1.26587967123436e-08 35270.9060434889 -730007.231586691;-0.000525 1.25001164640264e-08 55894.5318044012 -728718.331977109;-0.00045 1.2331443813866e-08 76473.4763318042 -726846.906082708;-0.000375 1.21529135961982e-08 96991.2891323108 -724394.449892715;-0.0003 1.19646685253474e-08 117431.568580302 -721362.923863085;-0.000225 1.1766859081543e-08 137777.975029133 -717754.751349341;-0.00015 1.15596433906279e-08 158014.243872799 -713572.816669385;-7.5e-05 1.13431870976547e-08 178124.198547612 -708820.462797813]  x3=[-0.002325 3.49648967161325e-12 0 0;-0.00225 3.99255046412127e-12 0 0;-0.002175 4.48541967287634e-12 0 0;-0.0021 4.97470330577413e-12 0 0;-0.002025 5.4600102369648e-12 0 0;-0.00195 5.94095251951299e-12 0 0;-0.001875 6.41714569551671e-12 0 0;-0.0018 6.88820910343706e-12 0 0;-0.001725 7.35376618239325e-12 0 0;-0.00165 7.81344477317963e-12 0 0;-0.001575 8.26687741576405e-12 0 0;-0.0015 8.71370164302977e-12 0 0;-0.001425 9.15356027052616e-12 -163.959464483953 -404.071950170932;-0.00135 9.58610168199646e-12 -152.470711052387 -408.545860688619;-0.001275 1.00109801104544e-11 -140.860074867286 -412.693185896232;-0.0012 1.04278559145853e-11 -129.136837293568 -416.510610485457;-0.001125 1.08363958502495e-11 -117.310369707977 -419.995082865486;-0.00105 1.12362733368735e-11 -105.390126007751 -423.143817602413;-0.000975 1.16271687185127e-11 -93.3856350533166 -425.954297645866;-0.0009 1.200876951938e-11 -81.306493051069 -428.4242763411;-0.000825 1.23807706936338e-11 -69.1623558823074 -430.551779224939;-0.00075 1.27428748692273e-11 -56.962931384473 -432.335105604128;-0.000675 1.30947925856229e-11 -44.7179715908519 -433.772829914846;-0.0006 1.34362425251825e-11 -32.437264934949 -434.863802862277;-0.000525 1.37669517380489e-11 -20.1306284257639 -435.607152339339;-0.00045 1.40866558603374e-11 -7.80789980022419 -436.002284123834;-0.000375 1.43950993254642e-11 4.52107034095093 -436.048882353459;-0.0003 1.46920355684425e-11 16.8464264076702 -435.746909778302;-0.000225 1.49772272229832e-11 29.1583156988782 -435.09660779062;-0.00015 1.52504463112411e-11 41.4468962786536 -434.098496231871;-7.5e-05 1.55114744260574e-11 53.7023448437027 -432.753372977165]  x4=[-0.002325 1.5099725145416e-11 0 0;-0.00225 1.49934491102579e-11 0 0;-0.002175 1.48751875412885e-11 0 0;-0.0021 1.47450349749966e-11 0 0;-0.002025 1.46030954533522e-11 0 0;-0.00195 1.44494824406374e-11 0 0;-0.001875 1.42843187327439e-11 0 0;-0.0018 1.41077363590129e-11 0 0;-0.001725 1.39198764766922e-11 0 0;-0.00165 1.37208892580972e-11 0 0;-0.001575 1.35109337705659e-11 0 0;-0.0015 1.32901778493027e-11 0 0;-0.001425 1.30587979632133e-11 -1447.81766818151 -4750.17763764101;-0.00135 1.28169790738384e-11 -1312.94851541751 -4789.20959204488;-0.001275 1.25649144874982e-11 -1177.02981169907 -4824.41312557824;-0.0012 1.23028057007663e-11 -1040.17020835832 -4855.76009707501;-0.001125 1.20308622393965e-11 -902.479108868145 -4883.2254482458;-0.00105 1.17493014908309e-11 -764.066581386735 -4906.78722370911;-0.000975 1.14583485304239e-11 -625.043270770775 -4926.42658854216;-0.0009 1.11582359415202e-11 -485.520310127644 -4942.12784333718;-0.000825 1.08492036295317e-11 -345.609231977307 -4953.87843675132;-0.00075 1.053149863016e-11 -205.421879094925 -4961.66897554001;-0.000675 1.02053749119208e-11 -65.0703151054552 -4965.49323206573;-0.0006 9.87109317312441e-12 75.3332650983007 -4965.34814927633;-0.000525 9.52892063347823e-12 215.676625042575 -4961.23384314878;-0.00045 9.17913082047504e-12 355.847576392753 -4953.15360259644;-0.000375 8.82200335073936e-12 495.734068635012 -4941.11388683997;-0.0003 8.45782370650628e-12 635.224278647791 -4925.12432024394;-0.000225 8.08688300741126e-12 774.206700091476 -4905.19768462324;-0.00015 7.70947777777358e-12 912.570232544868 -4881.34990902549;-7.5e-05 7.32590970955931e-12 1050.20427031716 -4853.60005699762]  x5=0.00231306500901259  V1=ones(3,3)  V2=ones(3,3)  I1=ones(3,3)  I2=ones(3,3)  nHarmo=1  Measurements=None  Decoupling=on  VsMag0=[602176.30241448 602177.107483122 602176.165721077]  VrMag0=[596743.737336293 596743.911083344 596743.706580488]  VsAngle0=[11.6043495452494 -108.395709698226 131.604253585455]  VrAngle0=[-14.2738568821762 -134.273869923445 105.726122150017]  IsMag0=[359.48626515744 359.489496854299 359.49191879915]  IrMag0=[4093.84062560465 4093.84102057892 4093.83505039196]  IsAngle0=[-21.3064747487055 -141.305731641511 98.6934507450505]  IrAngle0=[-16.1707432095149 -136.170836500553 103.829205357652]
      settings: AttributesFormatString=\n  LibrarySourceBlock=sps_lib/Power Grid Elements/Distributed Parameters Line
  MIC-MAN 60 km : spsDistributedParametersLineLib/Distributed Parameters Line  Phases=3  Length=60  Frequency=60  Resistance="[0.01273  0.3864]"  Inductance="[0.9337e-3  4.1264e-3]"  Capacitance=[12.74e-9 7.751e-9]  x1=[-0.000375 3.70689940758025e-09 367056.472396768 -647795.562768113;-0.0003 3.62309696526611e-09 385223.313915946 -637159.785534523;-0.000225 3.53639827467318e-09 403082.213812094 -626014.672517248;-0.00015 3.44687264140818e-09 420618.895953885 -614369.132949109;-7.5e-05 3.35459163089256e-09 437819.341785936 -602232.476096253]  x2=[-0.000375 1.14735724448663e-09 381674.19327137 -619636.360457307;-0.0003 1.09417101693894e-09 399039.114850723 -608598.586309297;-0.000225 1.04011012582169e-09 416085.050667168 -597074.307763262;-0.00015 9.85217786584077e-10 432798.374460424 -585072.737151144;-7.5e-05 9.29537879322206e-10 449165.725855173 -572603.46834486]  x3=[-0.000375 -8.43247484468703e-12 2615.73591803646 -3083.53120523905;-0.0003 -9.17875917917623e-12 2701.86358792149 -3008.35057124514;-0.000225 -9.91770615401733e-12 2785.83142939425 -2930.76510783387;-0.00015 -1.06487250663049e-11 2867.57231984699 -2850.83683563762;-7.5e-05 -1.13712315507054e-11 2947.02091686258 -2768.62964809422]  x4=[-0.000375 1.88537454353199e-11 -38.3285845652811 -1696.07516225759;-0.0003 1.9434099885982e-11 9.63578970452031 -1696.48092157581;-0.000225 1.99989190145468e-11 57.5924612714645 -1695.53054000236;-0.00015 2.05477513132452e-11 105.503094306062 -1693.22477725772;-7.5e-05 2.10801580539349e-11 153.329389781324 -1689.56547653334]  x5=0.000339324940197445  V1=ones(3,3)  V2=ones(3,3)  I1=ones(3,3)  I2=ones(3,3)  nHarmo=1  Measurements=None  Decoupling=on  VsMag0=[607930.231676026 607930.976808573 607930.152147035]  VrMag0=[594207.380493384 594208.101305747 594207.286862453]  VsAngle0=[7.63692875074031 -112.363120449614 127.636843332411]  VrAngle0=[9.73160889878888 -110.268441654022 129.731523430542]  IsMag0=[3306.19691878102 3306.20035207259 3306.19654855297]  IrMag0=[1387.14843174275 1387.1508825635 1387.14865267849]  IsAngle0=[18.4076953761245 -101.592346383779 138.407622969112]  IrAngle0=[-23.1945765462699 -143.1946244543 96.805311831549]
      settings: AttributesFormatString=\n  LibrarySourceBlock=sps_lib/Power Grid Elements/Distributed Parameters Line
  Regulateurs6 : Subsystem
  Regulateurs7 : Subsystem
  "MIC7a " : PMIOPort  Side=Left
  MIC7b : PMIOPort  Port=2  Side=Left
  MIC7c : PMIOPort  Port=3  Side=Left
  QUE7a : PMIOPort  Port=4  Side=Left
  QUE7b : PMIOPort  Port=5  Side=Left
  QUE7c : PMIOPort  Port=6  Side=Left
  wires:
  Regulateurs6/1(Pm) -> "B_6 CHU-5600 MVA "/1
  Regulateurs6/2(Vf) -> "B_6 CHU-5600 MVA "/2
  "B_6 CHU-5600 MVA "/1 -> Regulateurs6/1(m)
  Regulateurs7/1(Pm) -> B_7 MAN 5000 MVA/1
  Regulateurs7/2(Vf) -> B_7 MAN 5000 MVA/2
  B_7 MAN 5000 MVA/1 -> Regulateurs7/1(m)
  connections:
  "Cs PER "/RConn3 -- MIC-LTD 409 km/LConn3
  "Cs PER "/RConn2 -- MIC-LTD 409 km/LConn2
  "Cs PER "/RConn1 -- MIC-LTD 409 km/LConn1
  Cs BER/RConn3 -- MAN-LEV 3*379km/LConn3
  Cs BER/RConn2 -- MAN-LEV 3*379km/LConn2
  Cs BER/RConn1 -- MAN-LEV 3*379km/LConn1
  Cs ARNS2/RConn3 -- ARN-MAN 2*169km/LConn3
  Cs ARNS2/RConn2 -- ARN-MAN 2*169km/LConn2
  Cs ARNS2/RConn1 -- ARN-MAN 2*169km/LConn1
  CHU-ARN 3*450km/RConn3 -- "Cs MTG+ARNN "/LConn3
  CHU-ARN 3*450km/RConn2 -- "Cs MTG+ARNN "/LConn2
  CHU-ARN 3*450km/RConn1 -- "Cs MTG+ARNN "/LConn1
  Load Flow Bus2/LConn1 -- 5600 MVA 13.8 kV/735 kV1/RConn3 -- CHU-ARN 3*450km/LConn3 -- CHU 330 Mvar/LConn3
  5600 MVA 13.8 kV/735 kV1/RConn2 -- CHU-ARN 3*450km/LConn2 -- CHU 330 Mvar/LConn2
  5600 MVA 13.8 kV/735 kV1/RConn1 -- CHU-ARN 3*450km/LConn1 -- CHU 330 Mvar/LConn1
  "B_6 CHU-5600 MVA "/RConn3 -- Load Flow Bus1/LConn1 -- 5600 MVA 13.8 kV/735 kV1/LConn3 -- 280 MW/LConn3
  5600 MVA 13.8 kV/735 kV1/LConn2 -- "B_6 CHU-5600 MVA "/RConn2 -- 280 MW/LConn2
  5600 MVA 13.8 kV/735 kV1/LConn1 -- "B_6 CHU-5600 MVA "/RConn1 -- 280 MW/LConn1
  "Cs ARNS1 "/RConn1 -- ARN-MIC 180km/LConn1
  "Cs ARNS1 "/RConn2 -- ARN-MIC 180km/LConn2
  "Cs ARNS1 "/RConn3 -- ARN-MIC 180km/LConn3
  "Cs PER "/LConn3 -- Load Flow Bus6/LConn1 -- MIC7c/RConn1 -- MIC-MAN 60 km/LConn3 -- ARN-MIC 180km/RConn3
  "Cs PER "/LConn2 -- MIC7b/RConn1 -- ARN-MIC 180km/RConn2 -- MIC-MAN 60 km/LConn2
  "Cs PER "/LConn1 -- "MIC7a "/RConn1 -- ARN-MIC 180km/RConn1 -- MIC-MAN 60 km/LConn1
  ARN-MAN 2*169km/RConn1 -- MAN7/LConn1
  ARN-MAN 2*169km/RConn2 -- MAN7/LConn2
  ARN-MAN 2*169km/RConn3 -- MAN7/LConn3
  Cs BER/LConn1 -- 5000 MVA 13.8 kV/735 kV2/RConn1 -- MIC-MAN 60 km/RConn1 -- MAN-MIC 1650 Mvar/LConn1 -- MAN7/RConn1
  Cs BER/LConn2 -- 5000 MVA 13.8 kV/735 kV2/RConn2 -- MIC-MAN 60 km/RConn2 -- MAN-MIC 1650 Mvar/LConn2 -- MAN7/RConn2
  Cs BER/LConn3 -- Load Flow Bus5/LConn1 -- 5000 MVA 13.8 kV/735 kV2/RConn3 -- MIC-MAN 60 km/RConn3 -- MAN-MIC 1650 Mvar/LConn3 -- MAN7/RConn3
  B_7 MAN 5000 MVA/RConn1 -- 5000 MVA 13.8 kV/735 kV2/LConn1 -- 250 MW/LConn1
  B_7 MAN 5000 MVA/RConn2 -- 5000 MVA 13.8 kV/735 kV2/LConn2 -- 250 MW/LConn2
  B_7 MAN 5000 MVA/RConn3 -- 5000 MVA 13.8 kV/735 kV2/LConn3 -- Load Flow Bus3/LConn1 -- 250 MW/LConn3
  MIC-LTD 409 km/RConn2 -- MAN-LEV 3*379km/RConn2 -- QUE7b/RConn1
  Cs ARNS2/LConn1 -- ARN 990 Mvar/LConn1 -- "Cs MTG+ARNN "/RConn1 -- "Cs ARNS1 "/LConn1
  Cs ARNS2/LConn2 -- ARN 990 Mvar/LConn2 -- "Cs MTG+ARNN "/RConn2 -- "Cs ARNS1 "/LConn2
  Cs ARNS2/LConn3 -- Load Flow Bus4/LConn1 -- "Cs ARNS1 "/LConn3 -- ARN 990 Mvar/LConn3 -- "Cs MTG+ARNN "/RConn3
  MIC-LTD 409 km/RConn1 -- QUE7a/RConn1 -- MAN-LEV 3*379km/RConn1
  MIC-LTD 409 km/RConn3 -- QUE7c/RConn1 -- MAN-LEV 3*379km/RConn3
